simulink model "simulation"  (R2022b)
settings: Solver=VariableStepAuto  StartTime=0.0  StopTime=20  RelTol=1e-3
values from neighbouring files (symbols this model uses):
  A_new = double(subs(A, variables, values))    [Assignment_1.m]    (also in Group35_Assignment1.m)
  B_new = double(subs(B, variables, values))    [Assignment_1.m]    (also in Group35_Assignment1.m)
  C_new_a = double(subs(C_a, variables, values))    [Assignment_1.m]    (also in Group35_Assignment1.m)
  C_new_b = double(subs(C_b, variables, values))    [Assignment_1.m]    (also in Group35_Assignment1.m)
  D_new_a = double(subs(D_a, variables, values))    [Assignment_1.m]    (also in Group35_Assignment1.m)
  D_new_b = double(subs(D_b, variables, values))    [Assignment_1.m]    (also in Group35_Assignment1.m)
settings Model: Creator=soder  LastModifiedBy=soder

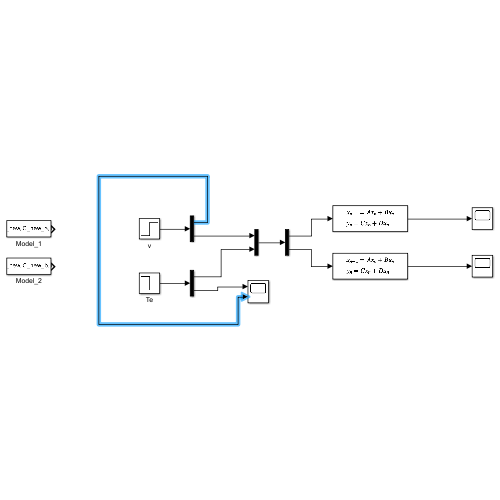
[thumbnail: Simulink's stored preview of the top-level diagram]
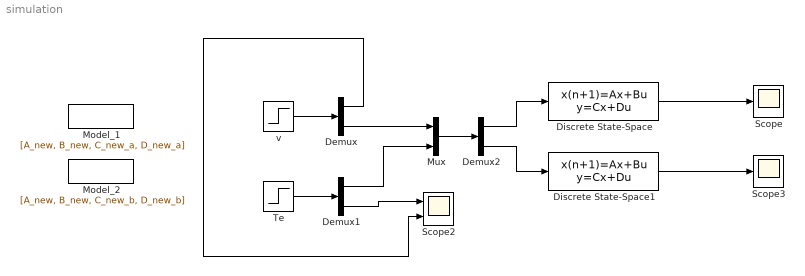
== system simulation ==
  Demux : Demux  Outputs=2
  Demux1 : Demux  Outputs=2
  Demux2 : Demux  Outputs=2
  Discrete State-Space : DiscreteStateSpace  A=A_new  B=B_new  C=C_new_a  D=D_new_a  SampleTime=-1
  Discrete State-Space1 : DiscreteStateSpace  A=A_new  B=B_new  C=C_new_b  D=D_new_b  SampleTime=-1
  Model_1 : FromWorkspace  VariableName=[A_new, B_new, C_new_a, D_new_a]
  Model_2 : FromWorkspace  VariableName=[A_new, B_new, C_new_b, D_new_b]
  Mux : Mux  Inputs=2
  Scope : Scope
  Scope2 : Scope  NumInputPorts=2
  Scope3 : Scope
  Te : Step  Time=10  After=-0.1  SampleTime=20
  v : Step  After=10  SampleTime=0
  wires:
  Discrete State-Space/1 -> Scope/1
  Te/1 -> Demux1/1
  Demux/2 -> Mux/1
  Mux/1 -> Demux2/1
  Demux2/1 -> Discrete State-Space/1
  Demux2/2 -> Discrete State-Space1/1
  Discrete State-Space1/1 -> Scope3/1
  Demux1/1 -> Mux/2
  Demux1/2 -> Scope2/1
  v/1 -> Demux/1
  Demux/1 -> Scope2/2
